simulink model "auction_with_real_uavs"  (R2022a)
settings: Solver=VariableStepAuto  StartTime=0.0  StopTime=120  RelTol=1e-3
settings Model: Creator=Kleber Cabral  LastModifiedBy=Kleber Cabral

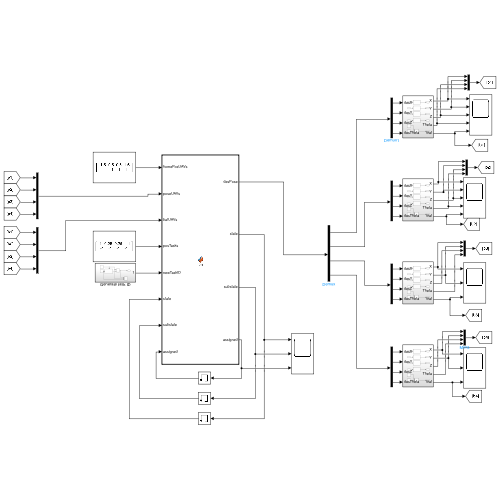
[thumbnail: Simulink's stored preview of the top-level diagram]
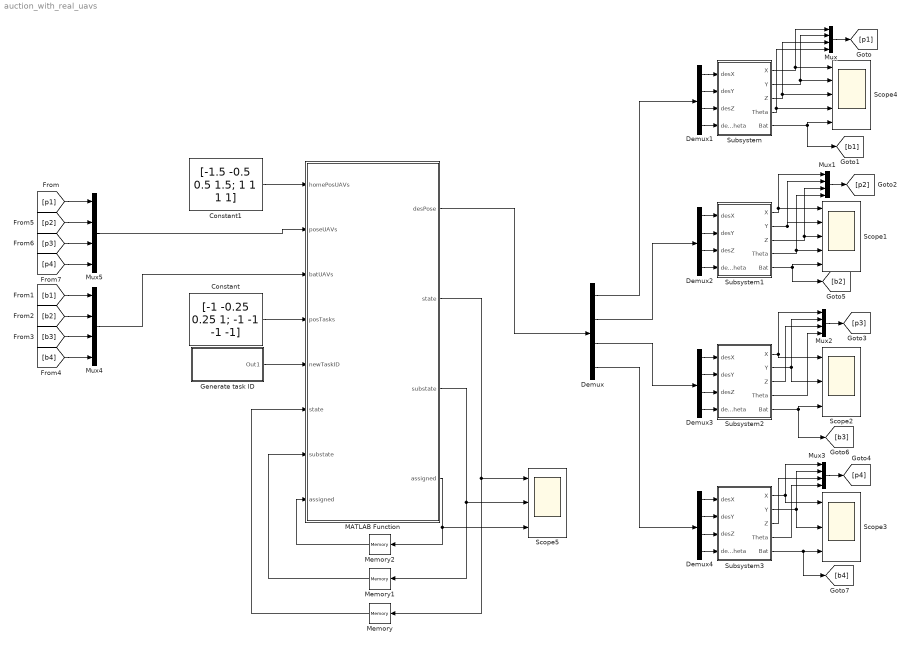
== system auction_with_real_uavs ==
  Constant : Constant  Value=[-1 -0.25 0.25 1; -1 -1 -1 -1]
  Constant1 : Constant  Value=[-1.5 -0.5 0.5 1.5; 1 1 1 1]
  Demux{,1..4} (5 alike) : Demux
  Generate task ID : Subsystem
  MATLAB Function : MATLAB Function  TreatAsAtomicUnit=on
  Memory : Memory  InitialCondition=1
  Memory1 : Memory  InitialCondition=1
  Memory2 : Memory  InitialCondition=[0 0 0 0]
  Mux{,1..5} (6 alike) : Mux
  Scope1 : Scope  NumInputPorts=5
  Scope2 : Scope  NumInputPorts=3
  Scope3 : Scope  NumInputPorts=3
  Scope4 : Scope  NumInputPorts=5
  Scope5 : Scope  NumInputPorts=3
  Subsystem : Subsystem
  Subsystem1 : Subsystem
  Subsystem2 : Subsystem
  Subsystem3 : Subsystem
  wires:
  Subsystem/1(X) -> Scope4/1, Mux/1
  Demux1/1 -> Subsystem/1(desX)
  Demux1/2 -> Subsystem/2(desY)
  Subsystem/5(Bat) -> Scope4/5, [b1]
  Subsystem1/5(Bat) -> Scope1/5, [b2]
  Subsystem2/5(Bat) -> Scope2/3, [b3]
  Subsystem3/5(Bat) -> [b4], Scope3/3
  Mux4/1 -> MATLAB Function/3(batUAVs)
  Mux/1 -> [p1]
  Mux1/1 -> [p2]
  Subsystem1/1(X) -> Mux1/1, Scope1/1
  Subsystem1/2(Y) -> Scope1/2, Mux1/2
  Subsystem2/2(Y) -> Scope2/2, Mux2/2
  Subsystem2/1(X) -> Scope2/1, Mux2/1
  Mux2/1 -> [p3]
  Mux3/1 -> [p4]
  Subsystem3/1(X) -> Scope3/1, Mux3/1
  Subsystem3/2(Y) -> Scope3/2, Mux3/2
  [p1] -> Mux5/1
  [b1] -> Mux4/1
  [b2] -> Mux4/2
  [b4] -> Mux4/4
  [b3] -> Mux4/3
  [p2] -> Mux5/2
  [p3] -> Mux5/3
  [p4] -> Mux5/4
  Mux5/1 -> MATLAB Function/2(poseUAVs)
  MATLAB Function/1(desPose) -> Demux/1
  Demux/1 -> Demux1/1
  Constant/1 -> MATLAB Function/4(posTasks)
  Constant1/1 -> MATLAB Function/1(homePosUAVs)
  Generate task ID/1(Out1) -> MATLAB Function/5(newTaskID)
  MATLAB Function/2(state) -> Scope5/1, Memory/1
  Memory/1 -> MATLAB Function/6("state ")
  MATLAB Function/3(substate) -> Scope5/2, Memory1/1
  Memory1/1 -> MATLAB Function/7("substate ")
  MATLAB Function/4(assigned) -> Scope5/3, Memory2/1
  Memory2/1 -> MATLAB Function/8("assigned ")
  Demux1/3 -> Subsystem/3(desZ)
  Demux1/4 -> Subsystem/4(desTheta)
  Subsystem/3(Z) -> Mux/3, Scope4/3
  Demux2/1 -> Subsystem1/1(desX)
  Demux2/2 -> Subsystem1/2(desY)
  Demux2/3 -> Subsystem1/3(desZ)
  Demux2/4 -> Subsystem1/4(desTheta)
  Demux3/1 -> Subsystem2/1(desX)
  Demux3/2 -> Subsystem2/2(desY)
  Demux3/3 -> Subsystem2/3(desZ)
  Demux3/4 -> Subsystem2/4(desTheta)
  Demux4/1 -> Subsystem3/1(desX)
  Demux4/2 -> Subsystem3/2(desY)
  Demux4/3 -> Subsystem3/3(desZ)
  Demux4/4 -> Subsystem3/4(desTheta)
  Demux/4 -> Demux4/1
  Demux/3 -> Demux3/1
  Demux/2 -> Demux2/1
  Subsystem1/3(Z) -> Scope1/3, Mux1/3
  Subsystem2/3(Z) -> Mux2/3
  Subsystem3/3(Z) -> Mux3/3
  Subsystem/4(Theta) -> Scope4/4, Mux/4
  Subsystem1/4(Theta) -> Scope1/4, Mux1/4
  Subsystem2/4(Theta) -> Mux2/4
  Subsystem3/4(Theta) -> Mux3/4
  Subsystem/2(Y) -> Scope4/2, Mux/2

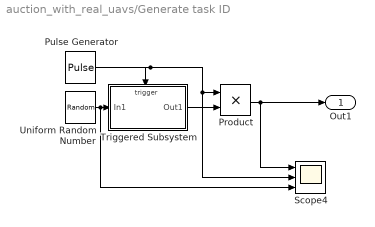
== system auction_with_real_uavs/Generate task ID ==
  Product : Product
  Pulse Generator : DiscretePulseGenerator  PulseType=Time based  Period=10  PulseWidth=0.1  PhaseDelay=30
  Scope4 : Scope  NumInputPorts=3
  Triggered Subsystem : Subsystem  TreatAsAtomicUnit=on
  Uniform Random Number : UniformRandomNumber  Minimum=0.5  Maximum=4.5  SampleTime=1
  Out1 : Outport
  wires:
  Triggered Subsystem/1(Out1) -> Product/2
  Product/1 -> Out1/1, Scope4/1
  Uniform Random Number/1 -> Scope4/3, Triggered Subsystem/1(In1)
  Pulse Generator/1 -> Scope4/2, Product/1, Triggered Subsystem/Trigger

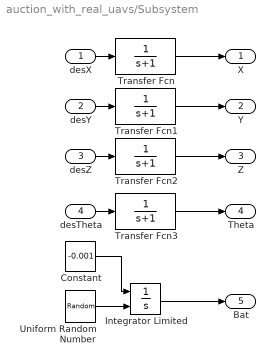
== system auction_with_real_uavs/Subsystem ==
  desX : Inport
  desY : Inport  Port=2
  desZ : Inport  Port=3
  desTheta : Inport  Port=4
  Constant : Constant  Value=-0.001
  Integrator Limited : Integrator  InitialConditionSource=external  InitialCondition=1  LimitOutput=on  UpperSaturationLimit=1  LowerSaturationLimit=0
  Transfer Fcn{,1..3} (4 alike) : TransferFcn  Denominator=[1 1]
  Uniform Random Number : UniformRandomNumber  Minimum=0.5  SampleTime=1
  X : Outport
  Y : Outport  Port=2
  Z : Outport  Port=3
  Theta : Outport  Port=4
  Bat : Outport  Port=5
  wires:
  desX/1 -> Transfer Fcn/1
  Constant/1 -> Integrator Limited/1
  Uniform Random Number/1 -> Integrator Limited/2
  Transfer Fcn/1 -> X/1
  desY/1 -> Transfer Fcn1/1
  Integrator Limited/1 -> Bat/1
  Transfer Fcn1/1 -> Y/1
  Transfer Fcn2/1 -> Z/1
  desZ/1 -> Transfer Fcn2/1
  desTheta/1 -> Transfer Fcn3/1
  Transfer Fcn3/1 -> Theta/1

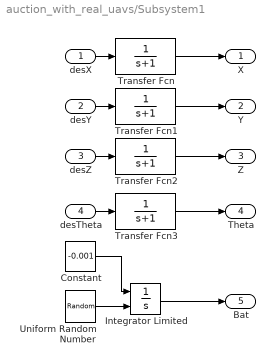
== system auction_with_real_uavs/Subsystem1 ==
  desX : Inport
  desY : Inport  Port=2
  desZ : Inport  Port=3
  desTheta : Inport  Port=4
  Constant : Constant  Value=-0.001
  Integrator Limited : Integrator  InitialConditionSource=external  InitialCondition=1  LimitOutput=on  UpperSaturationLimit=1  LowerSaturationLimit=0
  Transfer Fcn{,1..3} (4 alike) : TransferFcn  Denominator=[1 1]
  Uniform Random Number : UniformRandomNumber  Minimum=0.5  SampleTime=1
  X : Outport
  Y : Outport  Port=2
  Z : Outport  Port=3
  Theta : Outport  Port=4
  Bat : Outport  Port=5
  wires:
  Transfer Fcn3/1 -> Theta/1
  desTheta/1 -> Transfer Fcn3/1
  desZ/1 -> Transfer Fcn2/1
  Transfer Fcn2/1 -> Z/1
  Transfer Fcn1/1 -> Y/1
  Integrator Limited/1 -> Bat/1
  desY/1 -> Transfer Fcn1/1
  Transfer Fcn/1 -> X/1
  Uniform Random Number/1 -> Integrator Limited/2
  Constant/1 -> Integrator Limited/1
  desX/1 -> Transfer Fcn/1

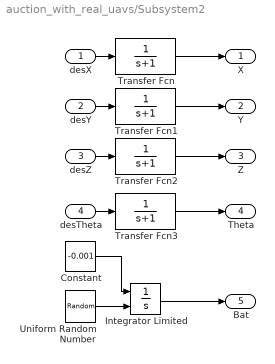
== system auction_with_real_uavs/Subsystem2 ==
  desX : Inport
  desY : Inport  Port=2
  desZ : Inport  Port=3
  desTheta : Inport  Port=4
  Constant : Constant  Value=-0.001
  Integrator Limited : Integrator  InitialConditionSource=external  InitialCondition=1  LimitOutput=on  UpperSaturationLimit=1  LowerSaturationLimit=0
  Transfer Fcn{,1..3} (4 alike) : TransferFcn  Denominator=[1 1]
  Uniform Random Number : UniformRandomNumber  Minimum=0.5  SampleTime=1
  X : Outport
  Y : Outport  Port=2
  Z : Outport  Port=3
  Theta : Outport  Port=4
  Bat : Outport  Port=5
  wires:
  desX/1 -> Transfer Fcn/1
  Constant/1 -> Integrator Limited/1
  Uniform Random Number/1 -> Integrator Limited/2
  Transfer Fcn/1 -> X/1
  desY/1 -> Transfer Fcn1/1
  Integrator Limited/1 -> Bat/1
  Transfer Fcn1/1 -> Y/1
  Transfer Fcn2/1 -> Z/1
  desZ/1 -> Transfer Fcn2/1
  desTheta/1 -> Transfer Fcn3/1
  Transfer Fcn3/1 -> Theta/1

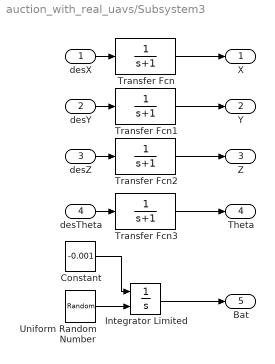
== system auction_with_real_uavs/Subsystem3 ==
  desX : Inport
  desY : Inport  Port=2
  desZ : Inport  Port=3
  desTheta : Inport  Port=4
  Constant : Constant  Value=-0.001
  Integrator Limited : Integrator  InitialConditionSource=external  InitialCondition=1  LimitOutput=on  UpperSaturationLimit=1  LowerSaturationLimit=0
  Transfer Fcn{,1..3} (4 alike) : TransferFcn  Denominator=[1 1]
  Uniform Random Number : UniformRandomNumber  Minimum=0.5  SampleTime=1
  X : Outport
  Y : Outport  Port=2
  Z : Outport  Port=3
  Theta : Outport  Port=4
  Bat : Outport  Port=5
  wires:
  Transfer Fcn3/1 -> Theta/1
  desTheta/1 -> Transfer Fcn3/1
  desZ/1 -> Transfer Fcn2/1
  Transfer Fcn2/1 -> Z/1
  Transfer Fcn1/1 -> Y/1
  Integrator Limited/1 -> Bat/1
  desY/1 -> Transfer Fcn1/1
  Transfer Fcn/1 -> X/1
  Uniform Random Number/1 -> Integrator Limited/2
  Constant/1 -> Integrator Limited/1
  desX/1 -> Transfer Fcn/1

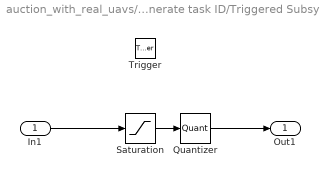
== system auction_with_real_uavs/Generate task ID/Triggered Subsystem ==
  In1 : Inport
  Trigger : TriggerPort  VariantControl=(inherit)
  Quantizer : Quantizer  QuantizationInterval=1
  Saturation : Saturate  UpperLimit=4  LowerLimit=1
  Out1 : Outport
  wires:
  In1/1 -> Saturation/1
  Saturation/1 -> Quantizer/1
  Quantizer/1 -> Out1/1

== matlab function auction_with_real_uavs/MATLAB Function ==
  data: homePosUAVs input; poseUAVs input; batUAVs input; desPose output; posTasks input; newTaskID input; state input size=1; substate input; state output; substate output; assigned output; assigned input
function [desPose, state, substate, assigned] = fcn(...
    homePosUAVs, poseUAVs, batUAVs,...
    posTasks, newTaskID, state,...
    substate, assigned)

%STATE CONDITIONS
IDLE = 1;
MOVE2TASK = 2;
EXECTASK = 3;
MOVE2HPOS = 4;
  
%SUB STATE CONDITIONS
MOVE2INTERMPOS = 1;
MOVE2FINALPOS  = 2;
DOTASK = 3;
FINISHTASK = 4;

posUAVs=reshape(poseUAVs, [], 4);
posUAVs(4,:)=[];

desPos = [homePosUAVs;ones(1,size(homePosUAVs,2))];

    
switch state
    case IDLE
        %Able to run a task if one exists

        %Create the nodes in space
        N=size(posUAVs,2);
        n=2;                % Variables of the state of each node
%         A = [0 1 1 1 1; 1 0 0 0 0; 1 0 0 0 0; 1 0 0 0 0; 1 0 0 0 0];
       
        assigned=assigned*0;

        if newTaskID > 0 % a new task has arrived 
            posTASK = posTasks(:,newTaskID);
            %computing graph and tree
%             G=graph(A);
%             pin=1;
%             [T.tree,T.parent] = minspantree(G,'Root',pin(1));
%     
            c=zeros(N,1);
            %Now, iteratively selects nodes from network
                
            %Compute the auction
            for i=1:N
                %each agend sends its bid
                c(i) = score(posUAVs(1:2,i), posTASK, batUAVs(i));
            end
            
            for i=1:N
                %discard invalid bids (not leaves and already assigned
                if assigned(i) > 0 
                    c(i) = 0;
                end
            end
            
%             if useRandomAsg
%                 winnerRand = randi(N);
%                 while c(winnerRand,idxAsgn)==0
%                     winnerRand = randi(N);
%                 end
%                 winner=winnerRand;
%             else
                [~,winner] = max(c); %maximum reward wins        
%             end
            
%             pos_winner=posUAVs(:,winner);
            desPos(2,winner) = posTASK(2); 
            assigned(winner)=newTaskID;        % which structure it moves to
        
            state=MOVE2TASK;
            substate=MOVE2INTERMPOS;
        end

    case MOVE2TASK 
        %A robot was assigned and has to move to a task position 
        [taskID, robotID] = max(assigned);
        posTASK = posTasks(:,taskID);
        switch substate
            case MOVE2INTERMPOS
                %moving to an intermediate position
                desPos(2,robotID) = posTASK(2);
                if norm( posUAVs(1:2,robotID) - desPos(1:2,robotID)) < 0.05
                    substate=MOVE2FINALPOS;
                end

            case MOVE2FINALPOS
                %moving to the task position
                desPos(1:2,robotID) = posTASK(1:2);
                if norm( posUAVs(1:2,robotID) - posTASK ) < 0.05
                    state=EXECTASK;
                    substate=DOTASK;
                end
        end

    case EXECTASK
        %The assigned robot has reached task location and must execute it
        [taskID, robotID] = max(assigned);
        posTASK = posTasks(:,taskID);
        %doing 1 by 1 because of size-mismatching error
        desPos(1:2,robotID) = posTASK(1:2);
        %desPos(2,robotID) = posTASK(2);
        switch substate
            case DOTASK
                %move down
                desPos(3,robotID) = 0.1;
                if norm( posUAVs(1:3,robotID) - desPos(1:3,robotID)) < 0.05
                    substate=FINISHTASK;
                end
            case FINISHTASK
                %move up
                if norm( posUAVs(1:3,robotID) - desPos(1:3,robotID)) < 0.05
                    state=MOVE2HPOS;
                    substate=MOVE2INTERMPOS;
                end
        end


    case MOVE2HPOS
        %The assigned robot must move back to its original position
        [taskID, robotID] = max(assigned);
        posTASK = posTasks(:,taskID);
        switch substate
            case MOVE2INTERMPOS
                %moving to an intermediate position
                desPos(2,robotID) = posTASK(2);
                if norm( posUAVs(1:2,robotID) - desPos(1:2,robotID)) < 0.05
                    substate=MOVE2FINALPOS;
                end

            case MOVE2FINALPOS
                %moving to the home position
                if norm( posUAVs(1:2,robotID) - homePosUAVs(1:2,robotID) ) < 0.05
                    state=IDLE;
                    substate=MOVE2INTERMPOS;
                end
        end

end
state=state(1);
desPose = reshape_pose_output(desPos(1,:),desPos(2,:),desPos(3,:),[0 0 0 0]);
% 
% if PLOTGRAPH 
%     hold on
%     grid on 
%     plot(posUAVs(1,pin),posUAVs(2,pin),'ko','MarkerSize',25,'Linewidth',1.5); %auctioneer
%     %Plotting structures
%     for j=1:length(posTasks)
% %         plot(posTasks(1,j),posTasks(2,j), 'rx', 'MarkerSize',10)
%     end
%     valid_bids=[];
%     axis equal
% end
% 
% if PLOTGRAPH
%     h=plot(G,'XData',x(1,:),'YData',x(2,:));
%     highlight(h,T.tree);
%     drawnow
%     pause(0.1);
% end

end

function cij = score(pos, posST, bat)

cij = 1/ norm(pos-posST) + 1/bat;

end

function pose_output = reshape_pose_output(X_all, Y_all, Z_all, Theta_all)
pose_output=reshape([X_all; Y_all; Z_all; Theta_all],16,1);

end
